simulink model "car_trailer_parking_model"  (R2024b)
settings: Solver=ode15s  StartTime=0.0  StopTime=5  FixedStep=1e-6  MaxStep=0.1  RelTol=1e-3  AbsTol=1e-6
undefined symbols (not defined in the file): Ion, Lithium, ref_traj_parking, ref_traj_reverse, ref_traj_straight
libraries: autolibshared x2, slpidlib x2, spsBatteryLib x1, spsDCMachineLib x1, spsGroundLib x1, spsFullBridgeMMCLib x1, spsPWMGenerator2LevelLib x1, vehdynlibeom x1, spsVariableCapacitorLib x1, spsVariableResistorLib x1, spspowerguiLib x1
(part 1 of 2)
settings Model: Creator=jesss  LastModifiedBy=jesss
settings SolverCC: MaxConsecutiveZCs=50  MaxConsecutiveMinStep=5  ZeroCrossControl=DisableAll
settings DataIOCC: SaveOutput=off  SignalLogging=off  SaveTime=off  ReturnWorkspaceOutputs=off
settings DebuggingCC: RTPrefix=none  StringTruncationChecking=none  AlgebraicLoopMsg=none  SignalResolutionControl=None  InheritedTsInSrcMsg=none  MultiTaskDSMMsg=none  MultiTaskCondExecSysMsg=none  MultiTaskRateTransMsg=warning  TasksWithSamePriorityMsg=none  SigSpecEnsureSampleTimeMsg=none  IntegerOverflowMsg=none  ParameterDowncastMsg=none  ParameterOverflowMsg=none  ParameterTunabilityLossMsg=none  FcnCallInpInsideContextMsg=warning  FrameProcessingCompatibilityMsg=none  UnknownTsInhSupMsg=none  NonCurrentReleaseOperatingPointMsg=warning  IntegerSaturationMsg=none
settings ModelReferenceCC: UpdateModelReferenceTargets=IfOutOfDate

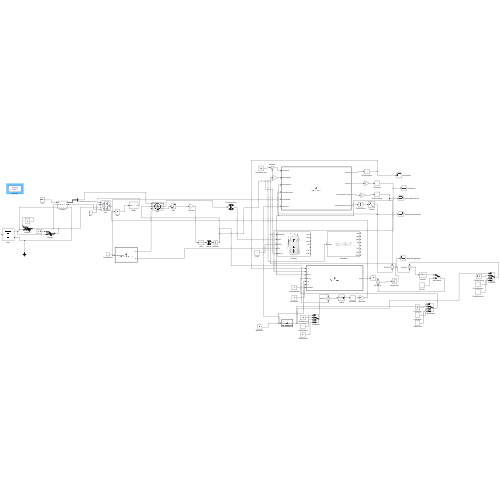
[thumbnail: Simulink's stored preview of the top-level diagram]
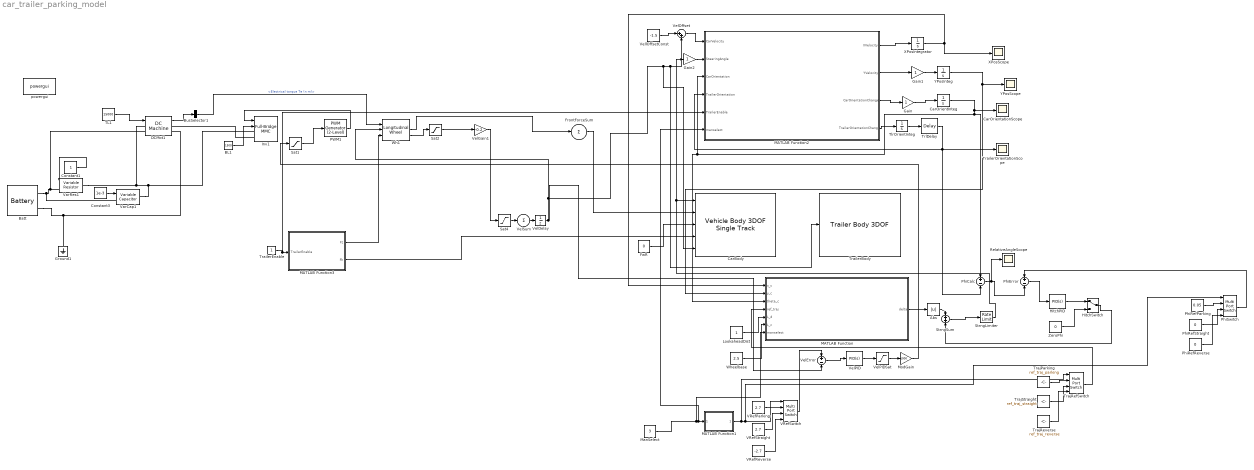
== system car_trailer_parking_model ==
  Abs : Abs  SaturateOnIntegerOverflow=off
  BL1 : Constant  Value=1500
  Batt : spsBatteryLib/Battery  BatType=Lithium-Ion  NomV=800  NomQ=100  SOC=100  Batt_Tr=0.01  PresetModel=on  MaxQ=100  MinV=600  FullV=931.1897  Dis_rate=43.4783  R=0.08  Normal_OP=90.4348  expZone="[864.3087      4.913043]"
  BusSelector1 : BusSelector  OutputSignals=Electrical torque Te (n m)
  CarBody : autolibshared/Vehicle Body 3DOF Single Track  trackMode=Single (bicycle)  inputMode=External longitudinal forces  frontSteerMode=on  rearSteerMode=off  windMode=off  muMode=off  extFMode=off  extMMode=off  htchFMode=on  htchMMode=off  extXo=off  extpsio=off  extxdoto=on  extro=off  extYo=off  extTamb=off  extydoto=off  aMode=2  NF=2  NR=2  m=3500  a=2  b=2  h=0.5  dh=1  hh=0.2  X_o=0  xdot_o=0  CalphaMode=off  sigmaMode=on  d=0  hl=0  w=[1.4,1.4]  Cy_f=100000  Cy_r=100000  sigma_f=0.3  sigma_r=0.3  alpha_f_brk=[-.1 .1]  Cy_f_data=[-9e3 9e3]  alpha_r_brk=[-.1 .1]  Cy_r_data=[-9e3 9e3]  Y_o=0  ydot_o=0  Izz=18667  psi_o=0  r_o=0  Af=2  Cd=0.3  Cl=0.1  Cpm=0  beta_w=[0 0.01:0.01:0.3]  Cs=[0 0.01:0.01:0.3]  Cym=[0 1e-6:0.01:0.3]  Pabs=101325  Tair=293  g=9.81  mu=0.8  xdot_tol=0.001  Fznom=8584  Fxtire_sat=7e4  Fytire_sat=7e4  longOff=0  latOff=0  vertOff=0  wrapAng=off
  CarOrientInteg : Integrator
  CarOrientationScope : Scope
  Constant1 : Constant
  Constant3 : Constant  Value=1e-3
  DCMot1 : spsDCMachineLib/DC Machine  PresetModel=No  MechanicalLoad=Torque TL  FieldType=Wound  ShowDetailedParameters=on  MeasurementBus=off  RLa="[0.8  0.01]"  RLf="[100  1]"  Laf=200  MachineConstant=Torque constant (N.m/A)  Ke=1.8  Kt=1.8  J=1000  Bm=0.01  Tf=0  w0=0  Ifinit=0  TsPowergui=0  TsBlock=-1
  FrontForceSum : Sum  Inputs=+
  FwR : Constant  Value=0
  Gain : Gain
  Gain1 : Gain
  Gain2 : Gain
  Ground1 : spsGroundLib/Ground  LConnTagsString=a
  HitchPID : slpidlib/PID Controller  Controller=PID  Form=Parallel  TimeDomain=Continuous-time  UseExternalTs=off  SampleTime=-1  IntegratorMethod=Forward Euler  FilterMethod=Forward Euler  ControllerParametersSource=internal  P=5  I=0.5  UseKiTs=off  D=0.05  UseExternalDerivativeSource=off  N=100  UseFilter=on  TunerSelectOption=Transfer Function Based (PID Tuner App)  InitialConditionSource=internal  InitialConditionForIntegrator=0  InitialConditionForFilter=0  DifferentiatorICPrevScaledInput=0  ExternalReset=none  TrackingMode=off  Kt=1  LimitOutput=off  SatLimitsSource=internal  UpperSaturationLimit=inf  LowerSaturationLimit=-inf  LinearizeAsGain=on  AntiWindupMode=none  Kb=1  LimitIntegrator=off  UpperIntegratorSaturationLimit=inf  LowerIntegratorSaturationLimit=-inf  POutMin=[]  POutMax=[]  IOutMin=[]  IOutMax=[]  DOutMin=[]  DOutMax=[]  NOutMin=[]  NOutMax=[]  SumOutMin=[]  SumOutMax=[]  SaturationOutMin=[]  SaturationOutMax=[]  PParamMin=[]  PParamMax=[]  IParamMin=[]  IParamMax=[]  DParamMin=[]  DParamMax=[]  NParamMin=[]  NParamMax=[]  KbParamMin=[]  KbParamMax=[]  KtParamMin=[]  KtParamMax=[]  KbOutMin=[]  KbOutMax=[]  KtOutMin=[]  KtOutMax=[]  IntegratorOutMin=[]  IntegratorOutMax=[]  FilterOutMin=[]  FilterOutMax=[]  SumI1OutMin=[]  SumI1OutMax=[]  SumI2OutMin=[]  SumI2OutMax=[]  SumI3OutMin=[]  SumI3OutMax=[]  SumI4OutMin=[]  SumI4OutMax=[]  SumDOutMin=[]  SumDOutMax=[]  DifferentiatorOutMin=[]  DifferentiatorOutMax=[]  FilterDiffOutCoefMin=[]  FilterDiffOutCoefMax=[]  ReciprocalOutMin=[]  ReciprocalOutMax=[]  SumDenOutMin=[]  SumDenOutMax=[]  SumNumOutMin=[]  SumNumOutMax=[]  DivideOutMin=[]  DivideOutMax=[]  UdiffTsProdOutMin=[]  UdiffTsProdOutMax=[]  NTsProdOutMin=[]  NTsProdOutMax=[]  UintegralTsProdOutMin=[]  UintegralTsProdOutMax=[]  UngainTsProdOutMin=[]  UngainTsProdOutMax=[]  ClampingZeroOutDataTypeStr=Inherit: Inherit via back propagation  ClampingZeroOutMin=[]  ClampingZeroOutMax=[]  FilterDenConstantOutDataTypeStr=Inherit: Inherit via back propagation  FilterDenConstantOutMin=[]  FilterDenConstantOutMax=[]  PCopyOutDataTypeStr=Inherit: Inherit via back propagation  PCopyOutMin=[]  PCopyOutMax=[]  NCopyOutDataTypeStr=Inherit: Inherit via back propagation  NCopyOutMin=[]  NCopyOutMax=[]  IntegratorContinuousStateAttributes=''  IntegratorStateMustResolveToSignalObject=off  IntegratorRTWStateStorageClass=Auto  FilterContinuousStateAttributes=''  FilterStateMustResolveToSignalObject=off  FilterRTWStateStorageClass=Auto  ParallelPVariant=InternalParameters  IdealPVariant=Disabled  IVariant=InternalParameters  DVariant=InternalParameters  IntegratorVariant=Continuous  SatVariant=Disabled  AWVariant=Passthrough  PCopyVariant=Disabled  TRVariant=Disabled  FdbkBlocksVariant=Forward  IdealPFdbkVariant=Disabled  SatFdbkVariant=Disabled  DerivativeFilterVariant=ContFilter  NVariant=InternalParameters  NCopyVariant=Disabled  FilterICVariant=InternalICsFilter  IntegratorICVariant=InternalICs  ExternalResetVariant=Disabled  TRSumVariant=Passthrough  SumFdbkVariant=Disabled  SumVariant=Sum_PID  TsampFilterVariant=InternalTs  TsampNgainVariant=Passthrough  TsampIntegralVariant=Disabled_SignalSpec  ExternalSaturationOutDataTypeStr=Inherit: Same as second input  DerivativeSourceVariant=ErrorSignal  PreIntVariant=InternalPreInt
  HitchSwitch : ManualSwitch
  Inv1 : spsFullBridgeMMCLib/Full-Bridge MMC  ModelType=Switching devices  n=1  C=1e-3  Vc_Initial=0  Ron=0.01  Rs=1e6  Cs=1e-9  Ron_Diode=1e-3  Rs_Diode=1e6  Cs_Diode=inf  Vf_Diode=1e-3  Rs_CurrentSource=inf  Ts=10e-6
      settings: LibrarySourceBlock=sps_lib/Power Electronics/Full-Bridge MMC
  LookaheadDist : Constant
  MATLAB Function : MATLAB Function  TreatAsAtomicUnit=on
  MATLAB Function1 : MATLAB Function  TreatAsAtomicUnit=on
  MATLAB Function2 : MATLAB Function  TreatAsAtomicUnit=on
  MATLAB Function3 : MATLAB Function  TreatAsAtomicUnit=on
  ManSelect : Constant  Value=3
  ModGain : Gain  Gain=1000
  PWM1 : spsPWMGenerator2LevelLib/PWM Generator (2-Level)  ModulatorType=Single-phase full-bridge (4 pulses)  ModulatorMode=Unsynchronized  Fc=10000  Pc=0  nF=27  MinMax=[-1, 1]  SamplingTechnique=Symmetrical regular (single edge)  ModulatingSignals=off  m=0.8  Freq=60  Phase=0  Ts=1e-5  ShowCarrierOutport=off
  PhiCalc : Sum  Inputs=+-
  PhiError : Sum  Inputs=+-
  PhiRefParking : Constant  Value=0.05
  PhiRefReverse : Constant  Value=0
  PhiRefStraight : Constant  Value=0
  PhiSwitch : MultiPortSwitch  SaturateOnIntegerOverflow=off  InputSameDT=off
  RelativeAngleScope : Scope
  Sat1 : Saturate  UpperLimit=50000  LowerLimit=-50000
  Sat2 : Saturate  UpperLimit=6  LowerLimit=-6
  Sat4 : Saturate  UpperLimit=2.5  LowerLimit=-2.5
  StrngLimiter : RateLimiter  RisingSlewLimit=0.5  FallingSlewLimit=-0.5  SampleTimeMode=inherited
  StrngSum : Sum
  TL1 : Constant  Value=15000
  TlrOrientInteg : Integrator
  TrailerBody : vehdynlibeom/Trailer Body 3DOF  trackMode=Dual 2-axle  inputMode=External longitudinal velocity  frontSteerMode=off  middleSteerMode=off  rearSteerMode=off  windMode=off  muMode=off  extFMode=off  extMMode=off  FhtchFMode=off  FhtchMMode=off  RhtchFMode=off  RhtchMMode=off  extXo=off  extpsio=off  extxdoto=off  extro=off  extYo=off  extTamb=off  extydoto=off  aMode=2  NF=1  NM=2  NR=2  m=10000  a=3  b=4.5  c=3  h=0.5  dh_f=7.5  hh_f=0.6  dh_r=7.5  hh_r=0.6  X_o=0  xdot_o=0  Lcpm=0  CalphaMode=off  sigmaMode=on  d=0  hl_f=0  hl_r=0  w_f=0.1  w_m=1.82  w_r=2  w=[0.1 2]  Cy_f=1000  Cy_m=11e3  Cy_r=150000  sigma_f=0.1  sigma_m=.1  sigma_r=0.3  alpha_f_brk=[-.1 .1]  Cy_f_data=[-9e3 9e3]  alpha_m_brk=[-.1 .1]  Cy_m_data=[-9e3 9e3]  alpha_r_brk=[-.1 .1]  Cy_r_data=[-9e3 9e3]  Y_o=0  ydot_o=0  Izz=30000  psi_o=0  r_o=0  Af=3  Cd=0.4  Cl=0.1  Cpm=0  beta_w=[0:0.01:0.3]  Cs=[0:0.03:0.9]  Cym=[0:0.01:0.3]  Pabs=101325  Tair=293  g=9.81  mu=0.8  xdot_tol=0.001  Fznom=32700  Fxtire_sat=7e4  Fytire_sat=7e4  longOff=0  latOff=0  vertOff=0  wrapAng=off
  TrailerEnable : Constant
  TrailerOrientationScope : Scope
  TrajParking : Constant  Value=ref_traj_parking
  TrajRefSwitch : MultiPortSwitch  SaturateOnIntegerOverflow=off  InputSameDT=off
  TrajReverse : Constant  Value=ref_traj_reverse
  TrajStraight : Constant  Value=ref_traj_straight
  TrlDelay : TransportDelay  DelayTime=0.01  BufferSize=10240
  VRefParking : Constant  Value=2.7
  VRefReverse : Constant  Value=-2.7
  VRefStraight : Constant  Value=2.7
  VRefSwitch : MultiPortSwitch  SaturateOnIntegerOverflow=off  InputSameDT=off
  VarCap1 : spsVariableCapacitorLib/Variable Capacitor  methode=Backward Euler  Cabsmin=1e-9  Initialize=off  vC0=0  C0=1e-6  iC0=0
      settings: LibrarySourceBlock=sps_lib/Passives/Variable Capacitor
  VarRes1 : spsVariableResistorLib/Variable Resistor  Rabsmin=1e-6
      settings: LibrarySourceBlock=sps_lib/Passives/Variable Resistor
  VelDelay : UnitDelay  SampleTime=1e-3  HasFrameUpgradeWarning=on
  VelError : Sum  Inputs=+-
  VelGain1 : Gain  Gain=-0.2
  VelOffset : Sum  Inputs=|++
  VelPID : slpidlib/PID Controller  Controller=PID  Form=Parallel  TimeDomain=Continuous-time  UseExternalTs=off  SampleTime=-1  IntegratorMethod=Forward Euler  FilterMethod=Forward Euler  ControllerParametersSource=internal  P=500  I=0.1  UseKiTs=off  D=0.2  UseExternalDerivativeSource=off  N=100  UseFilter=on  TunerSelectOption=Transfer Function Based (PID Tuner App)  InitialConditionSource=internal  InitialConditionForIntegrator=0  InitialConditionForFilter=0  DifferentiatorICPrevScaledInput=0  ExternalReset=none  TrackingMode=off  Kt=1  LimitOutput=on  SatLimitsSource=internal  UpperSaturationLimit=inf  LowerSaturationLimit=-inf  LinearizeAsGain=on  AntiWindupMode=back-calculation  Kb=1  LimitIntegrator=off  UpperIntegratorSaturationLimit=inf  LowerIntegratorSaturationLimit=-inf  POutMin=[]  POutMax=[]  IOutMin=[]  IOutMax=[]  DOutMin=[]  DOutMax=[]  NOutMin=[]  NOutMax=[]  SumOutMin=[]  SumOutMax=[]  SaturationOutMin=[]  SaturationOutMax=[]  PParamMin=[]  PParamMax=[]  IParamMin=[]  IParamMax=[]  DParamMin=[]  DParamMax=[]  NParamMin=[]  NParamMax=[]  KbParamMin=[]  KbParamMax=[]  KtParamMin=[]  KtParamMax=[]  KbOutMin=[]  KbOutMax=[]  KtOutMin=[]  KtOutMax=[]  IntegratorOutMin=[]  IntegratorOutMax=[]  FilterOutMin=[]  FilterOutMax=[]  SumI1OutMin=[]  SumI1OutMax=[]  SumI2OutMin=[]  SumI2OutMax=[]  SumI3OutMin=[]  SumI3OutMax=[]  SumI4OutMin=[]  SumI4OutMax=[]  SumDOutMin=[]  SumDOutMax=[]  DifferentiatorOutMin=[]  DifferentiatorOutMax=[]  FilterDiffOutCoefMin=[]  FilterDiffOutCoefMax=[]  ReciprocalOutMin=[]  ReciprocalOutMax=[]  SumDenOutMin=[]  SumDenOutMax=[]  SumNumOutMin=[]  SumNumOutMax=[]  DivideOutMin=[]  DivideOutMax=[]  UdiffTsProdOutMin=[]  UdiffTsProdOutMax=[]  NTsProdOutMin=[]  NTsProdOutMax=[]  UintegralTsProdOutMin=[]  UintegralTsProdOutMax=[]  UngainTsProdOutMin=[]  UngainTsProdOutMax=[]  ClampingZeroOutDataTypeStr=Inherit: Inherit via back propagation  ClampingZeroOutMin=[]  ClampingZeroOutMax=[]  FilterDenConstantOutDataTypeStr=Inherit: Inherit via back propagation  FilterDenConstantOutMin=[]  FilterDenConstantOutMax=[]  PCopyOutDataTypeStr=Inherit: Inherit via back propagation  PCopyOutMin=[]  PCopyOutMax=[]  NCopyOutDataTypeStr=Inherit: Inherit via back propagation  NCopyOutMin=[]  NCopyOutMax=[]  IntegratorContinuousStateAttributes=''  IntegratorStateMustResolveToSignalObject=off  IntegratorRTWStateStorageClass=Auto  FilterContinuousStateAttributes=''  FilterStateMustResolveToSignalObject=off  FilterRTWStateStorageClass=Auto  ParallelPVariant=InternalParameters  IdealPVariant=Disabled  IVariant=InternalParameters  DVariant=InternalParameters  IntegratorVariant=Continuous  SatVariant=Enabled  AWVariant=BackCalculation  PCopyVariant=Disabled  TRVariant=Disabled  FdbkBlocksVariant=Forward  IdealPFdbkVariant=Disabled  SatFdbkVariant=Disabled  DerivativeFilterVariant=ContFilter  NVariant=InternalParameters  NCopyVariant=Disabled  FilterICVariant=InternalICsFilter  IntegratorICVariant=InternalICs  ExternalResetVariant=Disabled  TRSumVariant=Passthrough  SumFdbkVariant=Disabled  SumVariant=Sum_PID  TsampFilterVariant=InternalTs  TsampNgainVariant=Passthrough  TsampIntegralVariant=Disabled_SignalSpec  ExternalSaturationOutDataTypeStr=Inherit: Same as second input  DerivativeSourceVariant=ErrorSignal  PreIntVariant=InternalPreInt
  VelPIDSat : Saturate  UpperLimit=50  LowerLimit=-50
  VelSum : Sum  Inputs=+
  VellOffsetConst : Constant  Value=-1.5
  Wh1 : autolibshared/Longitudinal Wheel  FxType=Magic Formula constant value  rollingType=None  BrakeType=None  vertType=None  lam_x=1  extMu=off  aMode=2  br=0  Iyy=5000  omegao=0  Lrel=0.3  Re=0.3  UNLOADED_RADIUS=0.4  LONGVL=16  gamma=0  NOMPRES=220000  press=220000  extPress=off  Dx=1  Cx=1.5  Bx=15  Ex=2  PCX1=1.6  PDX1=1  PDX2=-0.08  PDX3=0  PEX1=0.112  PEX2=0.313  PEX3=0  PEX4=0.0016  PKX1=21.7  PKX2=13.77  PKX3=-0.412  PHX1=2.1585E-4  PHX2=0.00115  PVX1=1.5973E-5  PVX2=1.043E-4  PPX1=-0.3489  PPX2=0.382  PPX3=-0.09634  PPX4=0.06447  lam_muV=1  lam_Kxkappa=1  lam_Cx=1  lam_Ex=0  lam_Hx=1  lam_Vx=1  kappaFx=[-1,-0.78476,-0.61585,-0.48329,-0.37927,-0.29764,-0.23357,-0.1833,-0.14384,-0.11288,-0.088587,-0.069519,-0.054556,-0.042813,-0.033598,-0.026367,-0.020691,-0.016238,-0.012743,-0.01,0.01,0.012743,0.016238,0.020691,0.026367,0.033598,0.042813,0.054556,0.069519,0.088587,0.11288,0.14384,0.1833,0.23357,0.29764,0.37927,0.48329,0.61585,0.78476,1]  FzFx=[0,200,400,600,800,1000,1200,1400,1600,1800,2000,2200,2400,2600,2800,3000,3200,3400,3600,3800,4000,4200,4400,4600,4800,5000,5200,5400,5600,5800,6000,6200,6400,6600,6800,7000,7200,7400,7600,7800,8000,8200,8400,8600,8800,9000,9200,9400,9600,9800,10000]  FxMap=|  aMy=84e-4  bMy=6.2e-4  cMy=1.6e-4  alphaMy=-0.003  betaMy=0.97  QSY1=0.007  QSY2=0  QSY3=0.0015  QSY4=8.5e-05  QSY5=0  QSY6=0  QSY7=0.9  QSY8=-0.4  lam_My=1  VxMy=-20:1:20  FzMy=0:200:1e4  MyMap=|  Fpl=10  Cr=1e-3  Kt=.008  Tmeas=25  Tamb=298.15  extTamb=off  mu_static=0.3  mu_kinetic=0.2  disk_abore=0.05  Rm=0.1778  num_pads=2  drum_abore=0.0508  drum_a=0.123  drum_c=0.212  drum_r=0.15  drum_theta1=0  drum_theta2=126  brake_p_bpt=[1 11.4736842105263 21.9473684210526 32.4210526315789 42.8947368421053 53.3684210526316 63.8421052631579 74.3157894736842 84.7894736842105 95.2631578947368 105.736842105263 116.210526315789 126.684210526316 137.157894736842 147.631578947368 158.105263157895 168.578947368421 179.052631578947 189.526315789474 200]  brake_n_bpt=[0 52.6315789473684 105.263157894737 157.894736842105 210.526315789474 263.157894736842 315.789473684211 368.421052631579 421.052631578947 473.684210526316 526.315789473684 578.947368421053 631.578947368421 684.210526315789 736.842105263158 789.473684210526 842.105263157895 894.736842105263 947.368421052632 1000]  f_brake_t=[43.4900602404453 42.5056030554862 41.5350898940194 40.5780454442085 39.6340111501808 38.7025443887544 37.7832176914519 36.8756180088306 35.9793460143796 35.0940154454303 34.2192524787115 33.3546951383474 32.4999927342521 31.6548053290159 30.8188032315107 29.991666515561 29.1730845621415 28.362755623661 27.5603864089927 26.765691687993;498.991217495636 487.695866636631 476.560505099801 465.579679307235 454.748127933653 444.060772460445 433.51270824929 423.099196101319 412.81565427025 402.657650900201 392.620896861006 382.701238955775 372.894653477208 363.197240090814 353.605216024701 344.114910546964 334.722759712992 325.425301366216 316.219170376863 307.10109410434;954.492374750826 932.886130217776 911.585920305583 890.581313170261 869.862244717126 849.419000532136 829.242198807128 809.322774193808 789.651962526121 770.221286354971 751.0225412433 732.047782773203 713.289314220164 694.739674852612 676.391628817892 658.238154578366 640.272434863842 622.48784710877 604.877954344734 587.436496520688;1409.99353200602 1378.07639379892 1346.61133551136 1315.58294703329 1284.9763615006 1254.77722860383 1224.97168936497 1195.5463522863 1166.48827078199 1137.78492180974 1109.42418562559 1081.39432659063 1053.68397496312 1026.28210961441 999.178041611083 972.361398609768 945.822110014692 919.550392851325 893.536738312604 867.771898937035;1865.49468926121 1823.26665738007 1781.63675071715 1740.58458089631 1700.09047828407 1660.13545667552 1620.7011799228 1581.76993037878 1543.32457903786 1505.34855726451 1467.82583000789 1430.74087040806 1394.07863570608 1357.82454437621 1321.96445440427 1286.48464264117 1251.37178516554 1216.61293859388 1182.19552228048 1148.10730135338;2320.9958465164 2268.45692096121 2216.66216592293 2165.58621475934 2115.20459506754 2065.49368474721 2016.43067048064 1967.99350847127 1920.16088729373 1872.91219271928 1826.22747439018 1780.08741422549 1734.47329644903 1689.36697913801 1644.75086719747 1600.60788667257 1556.92146031639 1513.67548433643 1470.85430624835 1428.44270376973;2776.49700377159 2713.64718454235 2651.68758112871 2590.58784862237 2530.31871185102 2470.8519128189 2412.16016103848 2354.21708656376 2296.9971955496 2240.47582817405 2184.62911877248 2129.43395804292 2074.86795719199 2020.9094138998 1967.53727999066 1914.73113070398 1862.47113546724 1810.73803007899 1759.51309021622 1708.77810618608;3231.99816102678 3158.8374481235 3086.71299633449 3015.58948248539 2945.43282863449 2876.21014089059 2807.88965159632 2740.44066465625 2673.83350380547 2608.03946362882 2543.03076315477 2478.78050186034 2415.26261793494 2352.4518486616 2290.32369278385 2228.85437473538 2168.02081061809 2107.80057582154 2048.17187418409 1989.11350860242;3687.49931828197 3604.02771170464 3521.73841154027 3440.59111634842 3360.54694541796 3281.56836896228 3203.61914215416 3126.66424274874 3050.66981206134 2975.60309908359 2901.43240753707 2828.12704567777 2755.6572786779 2683.9942834234 2613.11010557704 2542.97761876678 2473.57048576894 2404.8631215641 2336.83065815196 2269.44891101877;4143.00047553716 4049.21797528579 3956.76382674606 3865.59275021144 3775.66106220143 3686.92659703397 3599.34863271199 3512.88782084123 3427.50612031721 3343.16673453836 3259.83405191936 3177.4735894952 3096.05193942085 3015.5367181852 2935.89651837023 2857.10086279818 2779.12016091979 2701.92566730665 2625.48944211983 2549.78431343512;4598.50163279235 4494.40823886693 4391.78924195184 4290.59438407447 4190.77517898491 4092.28482510566 3995.07812326983 3899.11139893372 3804.34242857308 3710.73036999313 3618.23569630166 3526.82013331263 3436.44660016381 3347.079152947 3258.68293116342 3171.22410682959 3084.66983607064 2998.98821304921 2914.1482260877 2830.11971585147;5054.00279004754 4939.59850244808 4826.81465715762 4715.59601793749 4605.88929576838 4497.64305317735 4390.80761382767 4285.3349770262 4181.17873682896 4078.2940054479 3976.63734068395 3876.16667713006 3776.84126090677 3678.62158770879 3581.46934395661 3485.34735086099 ...(+2764 chars)]  FNOMIN=2000  lam_Fzo=1  m=10  zo=0  zdoto=0  g=9.81  VERTICAL_STIFFNESS=209000.0  VERTICAL_DAMPING=50  Q_RE0=.99  Q_V1=0  Q_V2=0.047  Q_FZ1=0  Q_FZ2=15.4  Q_FCX=0.134  Q_FCY=.11  Q_CAM=0  PFZ1=0.71  Q_FCY2=-0.48  Q_CAM1=85.2  Q_CAM2=257.0  Q_CAM3=0.512  Q_FYS1=-204500.0  Q_FYS2=-60000  Q_FYS3=88211.7  BOTTOM_OFFST=.01  BOTTOM_STIFF=2000000  zFz=[0 .01 .1]  pFz=[10000 1000000]  Fzz=[0 1e3 1e4; 0 1e4 1e5]  zdotFz=[-20 0 20]  Fzzdot=[500 0 -500;250 0 -250]  Gndz=0  extGnd=off  FZMIN=1000  FZMAX=50000  PRESMIN=10000  PRESMAX=1000000  kappamax=0.005  VXLOW=0.01  TMIN=0  TMAX=400  blkID=0
      FxMap=|
      | [-0,-131.22,-262.44,-393.66,-524.88,-656.1,-787.32,-918.54,-1049.8,-1181,-1312.2,-1443.4,-1574.6,-1705.9,-1837.1,-1968.3,-2099.5,-2230.7,-2362,-2493.2,-2624.4,-2755.6,-2886.8,-3018.1,-3149.3,-3280.5,-3411.7,-3542.9,-3674.2,-3805.4,-3936.6,-4067.8,-4199,-4330.2,-4461.5,-4592.7,-4723.9,-4855.1,-4986.3,-5117.6,-5248.8,-5380,-5511.2,-5642.4,-5773.7,-5904.9,-6036.1,-6167.3,-6298.5,-6429.8,-6561
      | -0,-137.87,-275.75,-413.62,-551.49,-689.36,-827.24,-965.11,-1103,-1240.9,-1378.7,-1516.6,-1654.5,-1792.3,-1930.2,-2068.1,-2206,-2343.8,-2481.7,-2619.6,-2757.5,-2895.3,-3033.2,-3171.1,-3308.9,-3446.8,-3584.7,-3722.6,-3860.4,-3998.3,-4136.2,-4274,-4411.9,-4549.8,-4687.7,-4825.5,-4963.4,-5101.3,-5239.2,-5377,-5514.9,-5652.8,-5790.6,-5928.5,-6066.4,-6204.3,-6342.1,-6480,-6617.9,-6755.8,-6893.6
      | -0,-145.88,-291.75,-437.63,-583.5,-729.38,-875.25,-1021.1,-1167,-1312.9,-1458.8,-1604.6,-1750.5,-1896.4,-2042.3,-2188.1,-2334,-2479.9,-2625.8,-2771.6,-2917.5,-3063.4,-3209.3,-3355.1,-3501,-3646.9,-3792.8,-3938.6,-4084.5,-4230.4,-4376.3,-4522.1,-4668,-4813.9,-4959.8,-5105.6,-5251.5,-5397.4,-5543.3,-5689.1,-5835,-5980.9,-6126.8,-6272.6,-6418.5,-6564.4,-6710.3,-6856.1,-7002,-7147.9,-7293.8
      | -0,-155.26,-310.53,-465.79,-621.05,-776.32,-931.58,-1086.8,-1242.1,-1397.4,-1552.6,-1707.9,-1863.2,-2018.4,-2173.7,-2328.9,-2484.2,-2639.5,-2794.7,-2950,-3105.3,-3260.5,-3415.8,-3571.1,-3726.3,-3881.6,-4036.8,-4192.1,-4347.4,-4502.6,-4657.9,-4813.2,-4968.4,-5123.7,-5278.9,-5434.2,-5589.5,-5744.7,-5900,-6055.3,-6210.5,-6365.8,-6521.1,-6676.3,-6831.6,-6986.8,-7142.1,-7297.4,-7452.6,-7607.9,-7763.2
      | -0,-165.86,-331.71,-497.57,-663.43,-829.28,-995.14,-1161,-1326.9,-1492.7,-1658.6,-1824.4,-1990.3,-2156.1,-2322,-2487.8,-2653.7,-2819.6,-2985.4,-3151.3,-3317.1,-3483,-3648.8,-3814.7,-3980.6,-4146.4,-4312.3,-4478.1,-4644,-4809.8,-4975.7,-5141.5,-5307.4,-5473.3,-5639.1,-5805,-5970.8,-6136.7,-6302.5,-6468.4,-6634.3,-6800.1,-6966,-7131.8,-7297.7,-7463.5,-7629.4,-7795.2,-7961.1,-8127,-8292.8
      | -0,-177.09,-354.19,-531.28,-708.38,-885.47,-1062.6,-1239.7,-1416.8,-1593.8,-1770.9,-1948,-2125.1,-2302.2,-2479.3,-2656.4,-2833.5,-3010.6,-3187.7,-3364.8,-3541.9,-3719,-3896.1,-4073.2,-4250.3,-4427.4,-4604.5,-4781.5,-4958.6,-5135.7,-5312.8,-5489.9,-5667,-5844.1,-6021.2,-6198.3,-6375.4,-6552.5,-6729.6,-6906.7,-7083.8,-7260.9,-7438,-7615.1,-7792.1,-7969.2,-8146.3,-8323.4,-8500.5,-8677.6,-8854.7
      | -0,-187.84,-375.67,-563.51,-751.35,-939.18,-1127,-1314.9,-1502.7,-1690.5,-1878.4,-2066.2,-2254,-2441.9,-2629.7,-2817.5,-3005.4,-3193.2,-3381.1,-3568.9,-3756.7,-3944.6,-4132.4,-4320.2,-4508.1,-4695.9,-4883.7,-5071.6,-5259.4,-5447.3,-5635.1,-5822.9,-6010.8,-6198.6,-6386.4,-6574.3,-6762.1,-6949.9,-7137.8,-7325.6,-7513.5,-7701.3,-7889.1,-8077,-8264.8,-8452.6,-8640.5,-8828.3,-9016.1,-9204,-9391.8
      | -0,-196.25,-392.49,-588.74,-784.98,-981.23,-1177.5,-1373.7,-1570,-1766.2,-1962.5,-2158.7,-2354.9,-2551.2,-2747.4,-2943.7,-3139.9,-3336.2,-3532.4,-3728.7,-3924.9,-4121.2,-4317.4,-4513.6,-4709.9,-4906.1,-5102.4,-5298.6,-5494.9,-5691.1,-5887.4,-6083.6,-6279.9,-6476.1,-6672.3,-6868.6,-7064.8,-7261.1,-7457.3,-7653.6,-7849.8,-8046.1,-8242.3,-8438.6,-8634.8,-8831,-9027.3,-9223.5,-9419.8,-9616,-9812.3
      | -0,-199.97,-399.95,-599.92,-799.9,-999.87,-1199.8,-1399.8,-1599.8,-1799.8,-1999.7,-2199.7,-2399.7,-2599.7,-2799.6,-2999.6,-3199.6,-3399.6,-3599.5,-3799.5,-3999.5,-4199.5,-4399.4,-4599.4,-4799.4,-4999.4,-5199.3,-5399.3,-5599.3,-5799.2,-5999.2,-6199.2,-6399.2,-6599.1,-6799.1,-6999.1,-7199.1,-7399,-7599,-7799,-7999,-8198.9,-8398.9,-8598.9,-8798.9,-8998.8,-9198.8,-9398.8,-9598.8,-9798.7,-9998.7
      | -0,-196.87,-393.74,-590.6,-787.47,-984.34,-1181.2,-1378.1,-1574.9,-1771.8,-1968.7,-2165.5,-2362.4,-2559.3,-2756.2,-2953,-3149.9,-3346.8,-3543.6,-3740.5,-3937.4,-4134.2,-4331.1,-4528,-4724.8,-4921.7,-5118.6,-5315.4,-5512.3,-5709.2,-5906,-6102.9,-6299.8,-6496.6,-6693.5,-6890.4,-7087.2,-7284.1,-7481,-7677.8,-7874.7,-8071.6,-8268.5,-8465.3,-8662.2,-8859.1,-9055.9,-9252.8,-9449.7,-9646.5,-9843.4
      | -0,-186.02,-372.04,-558.06,-744.08,-930.1,-1116.1,-1302.1,-1488.2,-1674.2,-1860.2,-2046.2,-2232.2,-2418.3,-2604.3,-2790.3,-2976.3,-3162.3,-3348.4,-3534.4,-3720.4,-3906.4,-4092.4,-4278.5,-4464.5,-4650.5,-4836.5,-5022.5,-5208.6,-5394.6,-5580.6,-5766.6,-5952.6,-6138.7,-6324.7,-6510.7,-6696.7,-6882.7,-7068.7,-7254.8,-7440.8,-7626.8,-7812.8,-7998.8,-8184.9,-8370.9,-8556.9,-8742.9,-8928.9,-9115,-9301
      | -0,-168.44,-336.89,-505.33,-673.78,-842.22,-1010.7,-1179.1,-1347.6,-1516,-1684.4,-1852.9,-2021.3,-2189.8,-2358.2,-2526.7,-2695.1,-2863.5,-3032,-3200.4,-3368.9,-3537.3,-3705.8,-3874.2,-4042.7,-4211.1,-4379.5,-4548,-4716.4,-4884.9,-5053.3,-5221.8,-5390.2,-5558.6,-5727.1,-5895.5,-6064,-6232.4,-6400.9,-6569.3,-6737.8,-6906.2,-7074.6,-7243.1,-7411.5,-7580,-7748.4,-7916.9,-8085.3,-8253.7,-8422.2
      | -0,-146.7,-293.4,-440.1,-586.81,-733.51,-880.21,-1026.9,-1173.6,-1320.3,-1467,-1613.7,-1760.4,-1907.1,-2053.8,-2200.5,-2347.2,-2493.9,-2640.6,-2787.3,-2934,-3080.7,-3227.4,-3374.1,-3520.8,-3667.5,-3814.2,-3960.9,-4107.6,-4254.3,-4401,-4547.7,-4694.5,-4841.2,-4987.9,-5134.6,-5281.3,-5428,-5574.7,-5721.4,-5868.1,-6014.8,-6161.5,-6308.2,-6454.9,-6601.6,-6748.3,-6895,-7041.7,-7188.4,-7335.1
      | -0,-123.75,-247.49,-371.24,-494.99,-618.73,-742.48,-866.23,-989.98,-1113.7,-1237.5,-1361.2,-1485,-1608.7,-1732.5,-1856.2,-1980,-2103.7,-2227.4,-2351.2,-2474.9,-2598.7,-2722.4,-2846.2,-2969.9,-3093.7,-3217.4,-3341.2,-3464.9,-3588.7,-3712.4,-3836.2,-3959.9,-4083.7,-4207.4,-4331.1,-4454.9,-4578.6,-4702.4,-4826.1,-4949.9,-5073.6,-5197.4,-5321.1,-5444.9,-5568.6,-5692.4,-5816.1,-5939.9,-6063.6,-6187.3
      | -0,-101.91,-203.81,-305.72,-407.63,-509.53,-611.44,-713.35,-815.25,-917.16,-1019.1,-1121,-1222.9,-1324.8,-1426.7,-1528.6,-1630.5,-1732.4,-1834.3,-1936.2,-2038.1,-2140,-2241.9,-2343.9,-2445.8,-2547.7,-2649.6,-2751.5,-2853.4,-2955.3,-3057.2,-3159.1,-3261,-3362.9,-3464.8,-3566.7,-3668.6,-3770.5,-3872.5,-3974.4,-4076.3,-4178.2,-4280.1,-4382,-4483.9,-4585.8,-4687.7,-4789.6,-4891.5,-4993.4,-5095.3
      | -0,-82.514,-165.03,-247.54,-330.06,-412.57,-495.09,-577.6,-660.12,-742.63,-825.14,-907.66,-990.17,-1072.7,-1155.2,-1237.7,-1320.2,-1402.7,-1485.3,-1567.8,-1650.3,-1732.8,-1815.3,-1897.8,-1980.3,-2062.9,-2145.4,-2227.9,-2310.4,-2392.9,-2475.4,-2557.9,-2640.5,-2723,-2805.5,-2888,-2970.5,-3053,-3135.6,-3218.1,-3300.6,-3383.1,-3465.6,-3548.1,-3630.6,-3713.2,-3795.7,-3878.2,-3960.7,-4043.2,-4125.7
      | -0,-66.058,-132.12,-198.17,-264.23,-330.29,-396.35,-462.41,-528.46,-594.52,-660.58,-726.64,-792.7,-858.76,-924.81,-990.87,-1056.9,-1123,-1189,-1255.1,-1321.2,-1387.2,-1453.3,-1519.3,-1585.4,-1651.5,-1717.5,-1783.6,-1849.6,-1915.7,-1981.7,-2047.8,-2113.9,-2179.9,-2246,-2312,-2378.1,-2444.2,-2510.2,-2576.3,-2642.3,-2708.4,-2774.4,-2840.5,-2906.6,-2972.6,-3038.7,-3104.7,-3170.8,-3236.8,-3302.9
      | -0,-52.494,-104.99,-157.48,-209.98,-262.47,-314.97,-367.46,-419.95,-472.45,-524.94,-577.44,-629.93,-682.43,-734.92,-787.41,-839.91,-892.4,-944.9,-997.39,-1049.9,-1102.4,-1154.9,-1207.4,-1259.9,-1312.4,-1364.9,-1417.3,-1469.8,-1522.3,-1574.8,-1627.3,-1679.8,-1732.3,-1784.8,-1837.3,-1889.8,-1942.3,-1994.8,-2047.3,-2099.8,-2152.3,-2204.8,-2257.3,-2309.7,-2362.2,-2414.7,-2467.2,-2519.7,-2572.2,-2624.7
      | -0,-41.519,-83.039,-124.56,-166.08,-207.6,-249.12,-290.64,-332.15,-373.67,-415.19,-456.71,-498.23,-539.75,-581.27,-622.79,-664.31,-705.83,-747.35,-788.87,-830.39,-871.91,-913.42,-954.94,-996.46,-1038,-1079.5,-1121,-1162.5,-1204.1,-1245.6,-1287.1,-1328.6,-1370.1,-1411.7,-1453.2,-1494.7,-1536.2,-1577.7,-1619.3,-1660.8,-1702.3,-1743.8,-1785.3,-1826.8,-1868.4,-1909.9,-1951.4,-1992.9,-2034.4,-2076
      | -0,-32.742,-65.483,-98.225,-130.97,-163.71,-196.45,-229.19,-261.93,-294.67,-327.42,-360.16,-392.9,-425.64,-458.38,-491.12,-523.86,-556.61,-589.35,-622.09,-654.83,-687.57,-720.31,-753.06,-785.8,-818.54,-851.28,-884.02,-916.76,-949.5,-982.25,-1015,-1047.7,-1080.5,-1113.2,-1146,-1178.7,-1211.4,-1244.2,-1276.9,-1309.7,-1342.4,-1375.1,-1407.9,-1440.6,-1473.4,-1506.1,-1538.9,-1571.6,-1604.3,-1637.1
      | 0,32.742,65.483,98.225,130.97,163.71,196.45,229.19,261.93,294.67,327.42,360.16,392.9,425.64,458.38,491.12,523.86,556.61,589.35,622.09,654.83,687.57,720.31,753.06,785.8,818.54,851.28,884.02,916.76,949.5,982.25,1015,1047.7,1080.5,1113.2,1146,1178.7,1211.4,1244.2,1276.9,1309.7,1342.4,1375.1,1407.9,1440.6,1473.4,1506.1,1538.9,1571.6,1604.3,1637.1
      | 0,41.519,83.039,124.56,166.08,207.6,249.12,290.64,332.15,373.67,415.19,456.71,498.23,539.75,581.27,622.79,664.31,705.83,747.35,788.87,830.39,871.91,913.42,954.94,996.46,1038,1079.5,1121,1162.5,1204.1,1245.6,1287.1,1328.6,1370.1,1411.7,1453.2,1494.7,1536.2,1577.7,1619.3,1660.8,1702.3,1743.8,1785.3,1826.8,1868.4,1909.9,1951.4,1992.9,2034.4,2076
      | 0,52.494,104.99,157.48,209.98,262.47,314.97,367.46,419.95,472.45,524.94,577.44,629.93,682.43,734.92,787.41,839.91,892.4,944.9,997.39,1049.9,1102.4,1154.9,1207.4,1259.9,1312.4,1364.9,1417.3,1469.8,1522.3,1574.8,1627.3,1679.8,1732.3,1784.8,1837.3,1889.8,1942.3,1994.8,2047.3,2099.8,2152.3,2204.8,2257.3,2309.7,2362.2,2414.7,2467.2,2519.7,2572.2,2624.7
      | 0,66.058,132.12,198.17,264.23,330.29,396.35,462.41,528.46,594.52,660.58,726.64,792.7,858.76,924.81,990.87,1056.9,1123,1189,1255.1,1321.2,1387.2,1453.3,1519.3,1585.4,1651.5,1717.5,1783.6,1849.6,1915.7,1981.7,2047.8,2113.9,2179.9,2246,2312,2378.1,2444.2,2510.2,2576.3,2642.3,2708.4,2774.4,2840.5,2906.6,2972.6,3038.7,3104.7,3170.8,3236.8,3302.9
      | 0,82.514,165.03,247.54,330.06,412.57,495.09,577.6,660.12,742.63,825.14,907.66,990.17,1072.7,1155.2,1237.7,1320.2,1402.7,1485.3,1567.8,1650.3,1732.8,1815.3,1897.8,1980.3,2062.9,2145.4,2227.9,2310.4,2392.9,2475.4,2557.9,2640.5,2723,2805.5,2888,2970.5,3053,3135.6,3218.1,3300.6,3383.1,3465.6,3548.1,3630.6,3713.2,3795.7,3878.2,3960.7,4043.2,4125.7
      | 0,101.91,203.81,305.72,407.63,509.53,611.44,713.35,815.25,917.16,1019.1,1121,1222.9,1324.8,1426.7,1528.6,1630.5,1732.4,1834.3,1936.2,2038.1,2140,2241.9,2343.9,2445.8,2547.7,2649.6,2751.5,2853.4,2955.3,3057.2,3159.1,3261,3362.9,3464.8,3566.7,3668.6,3770.5,3872.5,3974.4,4076.3,4178.2,4280.1,4382,4483.9,4585.8,4687.7,4789.6,4891.5,4993.4,5095.3
      | 0,123.75,247.49,371.24,494.99,618.73,742.48,866.23,989.98,1113.7,1237.5,1361.2,1485,1608.7,1732.5,1856.2,1980,2103.7,2227.4,2351.2,2474.9,2598.7,2722.4,2846.2,2969.9,3093.7,3217.4,3341.2,3464.9,3588.7,3712.4,3836.2,3959.9,4083.7,4207.4,4331.1,4454.9,4578.6,4702.4,4826.1,4949.9,5073.6,5197.4,5321.1,5444.9,5568.6,5692.4,5816.1,5939.9,6063.6,6187.3
      | 0,146.7,293.4,440.1,586.81,733.51,880.21,1026.9,1173.6,1320.3,1467,1613.7,1760.4,1907.1,2053.8,2200.5,2347.2,2493.9,2640.6,2787.3,2934,3080.7,3227.4,3374.1,3520.8,3667.5,3814.2,3960.9,4107.6,4254.3,4401,4547.7,4694.5,4841.2,4987.9,5134.6,5281.3,5428,5574.7,5721.4,5868.1,6014.8,6161.5,6308.2,6454.9,6601.6,6748.3,6895,7041.7,7188.4,7335.1
      | 0,168.44,336.89,505.33,673.78,842.22,1010.7,1179.1,1347.6,1516,1684.4,1852.9,2021.3,2189.8,2358.2,2526.7,2695.1,2863.5,3032,3200.4,3368.9,3537.3,3705.8,3874.2,4042.7,4211.1,4379.5,4548,4716.4,4884.9,5053.3,5221.8,5390.2,5558.6,5727.1,5895.5,6064,6232.4,6400.9,6569.3,6737.8,6906.2,7074.6,7243.1,7411.5,7580,7748.4,7916.9,8085.3,8253.7,8422.2
      | 0,186.02,372.04,558.06,744.08,930.1,1116.1,1302.1,1488.2,1674.2,1860.2,2046.2,2232.2,2418.3,2604.3,2790.3,2976.3,3162.3,3348.4,3534.4,3720.4,3906.4,4092.4,4278.5,4464.5,4650.5,4836.5,5022.5,5208.6,5394.6,5580.6,5766.6,5952.6,6138.7,6324.7,6510.7,6696.7,6882.7,7068.7,7254.8,7440.8,7626.8,7812.8,7998.8,8184.9,8370.9,8556.9,8742.9,8928.9,9115,9301
      | 0,196.87,393.74,590.6,787.47,984.34,1181.2,1378.1,1574.9,1771.8,1968.7,2165.5,2362.4,2559.3,2756.2,2953,3149.9,3346.8,3543.6,3740.5,3937.4,4134.2,4331.1,4528,4724.8,4921.7,5118.6,5315.4,5512.3,5709.2,5906,6102.9,6299.8,6496.6,6693.5,6890.4,7087.2,7284.1,7481,7677.8,7874.7,8071.6,8268.5,8465.3,8662.2,8859.1,9055.9,9252.8,9449.7,9646.5,9843.4
      | 0,199.97,399.95,599.92,799.9,999.87,1199.8,1399.8,1599.8,1799.8,1999.7,2199.7,2399.7,2599.7,2799.6,2999.6,3199.6,3399.6,3599.5,3799.5,3999.5,4199.5,4399.4,4599.4,4799.4,4999.4,5199.3,5399.3,5599.3,5799.2,5999.2,6199.2,6399.2,6599.1,6799.1,6999.1,7199.1,7399,7599,7799,7999,8198.9,8398.9,8598.9,8798.9,8998.8,9198.8,9398.8,9598.8,9798.7,9998.7
      | 0,196.25,392.49,588.74,784.98,981.23,1177.5,1373.7,1570,1766.2,1962.5,2158.7,2354.9,2551.2,2747.4,2943.7,3139.9,3336.2,3532.4,3728.7,3924.9,4121.2,4317.4,4513.6,4709.9,4906.1,5102.4,5298.6,5494.9,5691.1,5887.4,6083.6,6279.9,6476.1,6672.3,6868.6,7064.8,7261.1,7457.3,7653.6,7849.8,8046.1,8242.3,8438.6,8634.8,8831,9027.3,9223.5,9419.8,9616,9812.3
      | 0,187.84,375.67,563.51,751.35,939.18,1127,1314.9,1502.7,1690.5,1878.4,2066.2,2254,2441.9,2629.7,2817.5,3005.4,3193.2,3381.1,3568.9,3756.7,3944.6,4132.4,4320.2,4508.1,4695.9,4883.7,5071.6,5259.4,5447.3,5635.1,5822.9,6010.8,6198.6,6386.4,6574.3,6762.1,6949.9,7137.8,7325.6,7513.5,7701.3,7889.1,8077,8264.8,8452.6,8640.5,8828.3,9016.1,9204,9391.8
      | 0,177.09,354.19,531.28,708.38,885.47,1062.6,1239.7,1416.8,1593.8,1770.9,1948,2125.1,2302.2,2479.3,2656.4,2833.5,3010.6,3187.7,3364.8,3541.9,3719,3896.1,4073.2,4250.3,4427.4,4604.5,4781.5,4958.6,5135.7,5312.8,5489.9,5667,5844.1,6021.2,6198.3,6375.4,6552.5,6729.6,6906.7,7083.8,7260.9,7438,7615.1,7792.1,7969.2,8146.3,8323.4,8500.5,8677.6,8854.7
      | 0,165.86,331.71,497.57,663.43,829.28,995.14,1161,1326.9,1492.7,1658.6,1824.4,1990.3,2156.1,2322,2487.8,2653.7,2819.6,2985.4,3151.3,3317.1,3483,3648.8,3814.7,3980.6,4146.4,4312.3,4478.1,4644,4809.8,4975.7,5141.5,5307.4,5473.3,5639.1,5805,5970.8,6136.7,6302.5,6468.4,6634.3,6800.1,6966,7131.8,7297.7,7463.5,7629.4,7795.2,7961.1,8127,8292.8
      | 0,155.26,310.53,465.79,621.05,776.32,931.58,1086.8,1242.1,1397.4,1552.6,1707.9,1863.2,2018.4,2173.7,2328.9,2484.2,2639.5,2794.7,2950,3105.3,3260.5,3415.8,3571.1,3726.3,3881.6,4036.8,4192.1,4347.4,4502.6,4657.9,4813.2,4968.4,5123.7,5278.9,5434.2,5589.5,5744.7,5900,6055.3,6210.5,6365.8,6521.1,6676.3,6831.6,6986.8,7142.1,7297.4,7452.6,7607.9,7763.2
      | 0,145.88,291.75,437.63,583.5,729.38,875.25,1021.1,1167,1312.9,1458.8,1604.6,1750.5,1896.4,2042.3,2188.1,2334,2479.9,2625.8,2771.6,2917.5,3063.4,3209.3,3355.1,3501,3646.9,3792.8,3938.6,4084.5,4230.4,4376.3,4522.1,4668,4813.9,4959.8,5105.6,5251.5,5397.4,5543.3,5689.1,5835,5980.9,6126.8,6272.6,6418.5,6564.4,6710.3,6856.1,7002,7147.9,7293.8
      | 0,137.87,275.75,413.62,551.49,689.36,827.24,965.11,1103,1240.9,1378.7,1516.6,1654.5,1792.3,1930.2,2068.1,2206,2343.8,2481.7,2619.6,2757.5,2895.3,3033.2,3171.1,3308.9,3446.8,3584.7,3722.6,3860.4,3998.3,4136.2,4274,4411.9,4549.8,4687.7,4825.5,4963.4,5101.3,5239.2,5377,5514.9,5652.8,5790.6,5928.5,6066.4,6204.3,6342.1,6480,6617.9,6755.8,6893.6
      | 0,131.22,262.44,393.66,524.88,656.1,787.32,918.54,1049.8,1181,1312.2,1443.4,1574.6,1705.9,1837.1,1968.3,2099.5,2230.7,2362,2493.2,2624.4,2755.6,2886.8,3018.1,3149.3,3280.5,3411.7,3542.9,3674.2,3805.4,3936.6,4067.8,4199,4330.2,4461.5,4592.7,4723.9,4855.1,4986.3,5117.6,5248.8,5380,5511.2,5642.4,5773.7,5904.9,6036.1,6167.3,6298.5,6429.8,6561]
      MyMap=|
      | [0,1114.7,4367.1,9707.2,17109,26554,38030,51524,67028,84533,1.0403e+05,1.2552e+05,1.4899e+05,1.7444e+05,2.0185e+05,2.3124e+05,2.6259e+05,2.959e+05,3.3117e+05,3.6839e+05,4.0756e+05,4.4868e+05,4.9174e+05,5.3675e+05,5.8369e+05,6.3257e+05,6.8338e+05,7.3613e+05,7.908e+05,8.474e+05,9.0593e+05,9.6638e+05,1.0288e+06,1.093e+06,1.1593e+06,1.2274e+06,1.2974e+06,1.3694e+06,1.4432e+06,1.519e+06,1.5967e+06,1.6763e+06,1.7578e+06,1.8412e+06,1.9265e+06,2.0137e+06,2.1028e+06,2.1938e+06,2.2867e+06,2.3815e+06,2.4782e+06
      | 0,1024.5,4013.8,8921.9,15725,24406,34953,47356,61605,77694,95616,1.1537e+05,1.3694e+05,1.6032e+05,1.8553e+05,2.1254e+05,2.4135e+05,2.7197e+05,3.0438e+05,3.3859e+05,3.7459e+05,4.1238e+05,4.5196e+05,4.9333e+05,5.3647e+05,5.814e+05,6.281e+05,6.7658e+05,7.2683e+05,7.7885e+05,8.3264e+05,8.8821e+05,9.4553e+05,1.0046e+06,1.0655e+06,1.1281e+06,1.1925e+06,1.2586e+06,1.3265e+06,1.3961e+06,1.4675e+06,1.5407e+06,1.6156e+06,1.6922e+06,1.7706e+06,1.8508e+06,1.9327e+06,2.0163e+06,2.1017e+06,2.1889e+06,2.2777e+06
      | 0,938.57,3677,8173.3,14405,22358,32020,43382,56436,71175,87593,1.0568e+05,1.2545e+05,1.4687e+05,1.6996e+05,1.947e+05,2.211e+05,2.4915e+05,2.7884e+05,3.1018e+05,3.4316e+05,3.7778e+05,4.1404e+05,4.5193e+05,4.9146e+05,5.3261e+05,5.754e+05,6.1981e+05,6.6584e+05,7.135e+05,7.6278e+05,8.1368e+05,8.6619e+05,9.2032e+05,9.7607e+05,1.0334e+06,1.0924e+06,1.153e+06,1.2152e+06,1.279e+06,1.3444e+06,1.4114e+06,1.48e+06,1.5502e+06,1.6221e+06,1.6955e+06,1.7705e+06,1.8471e+06,1.9254e+06,2.0052e+06,2.0866e+06
      | 0,856.81,3356.7,7461.3,13151,20411,29231,39603,51520,64974,79962,96478,1.1452e+05,1.3408e+05,1.5515e+05,1.7774e+05,2.0184e+05,2.2744e+05,2.5455e+05,2.8316e+05,3.1327e+05,3.4487e+05,3.7797e+05,4.1256e+05,4.4864e+05,4.8621e+05,5.2527e+05,5.6581e+05,6.0784e+05,6.5134e+05,6.9633e+05,7.4279e+05,7.9073e+05,8.4015e+05,8.9104e+05,9.4341e+05,9.9724e+05,1.0525e+06,1.1093e+06,1.1676e+06,1.2273e+06,1.2885e+06,1.3511e+06,1.4152e+06,1.4808e+06,1.5478e+06,1.6163e+06,1.6862e+06,1.7576e+06,1.8305e+06,1.9048e+06
      | 0,779.25,3052.9,6785.9,11960,18563,26585,36018,46856,59093,72724,87745,1.0415e+05,1.2194e+05,1.4111e+05,1.6165e+05,1.8357e+05,2.0685e+05,2.3151e+05,2.5753e+05,2.8491e+05,3.1365e+05,3.4376e+05,3.7522e+05,4.0803e+05,4.422e+05,4.7772e+05,5.1459e+05,5.5282e+05,5.9238e+05,6.333e+05,6.7556e+05,7.1916e+05,7.641e+05,8.1039e+05,8.5801e+05,9.0697e+05,9.5727e+05,1.0089e+06,1.0619e+06,1.1162e+06,1.1718e+06,1.2288e+06,1.2871e+06,1.3467e+06,1.4077e+06,1.47e+06,1.5336e+06,1.5985e+06,1.6648e+06,1.7324e+06
      | 0,705.9,2765.5,6147.1,10834,16816,24083,32628,42446,53531,65879,79486,94348,1.1046e+05,1.2783e+05,1.4643e+05,1.6629e+05,1.8738e+05,2.0972e+05,2.3329e+05,2.5809e+05,2.8413e+05,3.114e+05,3.399e+05,3.6962e+05,4.0058e+05,4.3276e+05,4.6616e+05,5.0078e+05,5.3662e+05,5.7369e+05,6.1197e+05,6.5146e+05,6.9218e+05,7.3411e+05,7.7725e+05,8.216e+05,8.6717e+05,9.1394e+05,9.6193e+05,1.0111e+06,1.0615e+06,1.1131e+06,1.1659e+06,1.22e+06,1.2752e+06,1.3316e+06,1.3892e+06,1.4481e+06,1.5081e+06,1.5693e+06
      | 0,636.76,2494.6,5545,9773.1,15169,21724,29432,38288,48287,59426,71700,85106,99642,1.153e+05,1.3209e+05,1.5e+05,1.6903e+05,1.8917e+05,2.1044e+05,2.3281e+05,2.563e+05,2.809e+05,3.066e+05,3.3342e+05,3.6134e+05,3.9037e+05,4.205e+05,4.5173e+05,4.8406e+05,5.1749e+05,5.5202e+05,5.8765e+05,6.2438e+05,6.622e+05,7.0111e+05,7.4112e+05,7.8223e+05,8.2442e+05,8.677e+05,9.1208e+05,9.5754e+05,1.0041e+06,1.0517e+06,1.1005e+06,1.1503e+06,1.2012e+06,1.2532e+06,1.3062e+06,1.3604e+06,1.4156e+06
      | 0,571.82,2240.2,4979.5,8776.4,13622,19508,26430,34383,43363,53365,64388,76427,89480,1.0355e+05,1.1862e+05,1.347e+05,1.5179e+05,1.6988e+05,1.8897e+05,2.0907e+05,2.3016e+05,2.5225e+05,2.7534e+05,2.9942e+05,3.2449e+05,3.5056e+05,3.7761e+05,4.0566e+05,4.3469e+05,4.6472e+05,4.9573e+05,5.2772e+05,5.607e+05,5.9467e+05,6.2961e+05,6.6554e+05,7.0245e+05,7.4034e+05,7.7921e+05,8.1906e+05,8.5989e+05,9.017e+05,9.4448e+05,9.8824e+05,1.033e+06,1.0787e+06,1.1254e+06,1.173e+06,1.2216e+06,1.2712e+06
      | 0,511.09,2002.3,4450.7,7844.3,12175,17436,23623,30732,38757,47698,57549,68310,79977,92548,1.0602e+05,1.204e+05,1.3567e+05,1.5184e+05,1.689e+05,1.8686e+05,2.0572e+05,2.2546e+05,2.4609e+05,2.6762e+05,2.9003e+05,3.1332e+05,3.3751e+05,3.6258e+05,3.8853e+05,4.1536e+05,4.4308e+05,4.7167e+05,5.0115e+05,5.3151e+05,5.6274e+05,5.9486e+05,6.2785e+05,6.6171e+05,6.9646e+05,7.3207e+05,7.6857e+05,8.0593e+05,8.4417e+05,8.8328e+05,9.2326e+05,9.6412e+05,1.0058e+06,1.0484e+06,1.0919e+06,1.1362e+06
      | 0,454.56,1780.8,3958.4,6976.8,10828,15508,21011,27333,34471,42422,51185,60755,71132,82313,94296,1.0708e+05,1.2066e+05,1.3505e+05,1.5022e+05,1.662e+05,1.8296e+05,2.0052e+05,2.1888e+05,2.3802e+05,2.5795e+05,2.7867e+05,3.0018e+05,3.2248e+05,3.4556e+05,3.6942e+05,3.9407e+05,4.1951e+05,4.4573e+05,4.7273e+05,5.0051e+05,5.2907e+05,5.5841e+05,5.8853e+05,6.1943e+05,6.5111e+05,6.8356e+05,7.168e+05,7.5081e+05,7.8559e+05,8.2115e+05,8.5749e+05,8.946e+05,9.3248e+05,9.7114e+05,1.0106e+06
      | 0,402.25,1575.9,3502.8,6173.8,9582.1,13723,18592,24187,30503,37540,45293,53762,62945,72839,83443,94756,1.0678e+05,1.195e+05,1.3293e+05,1.4707e+05,1.6191e+05,1.7745e+05,1.9368e+05,2.1062e+05,2.2826e+05,2.466e+05,2.6563e+05,2.8536e+05,3.0578e+05,3.269e+05,3.4872e+05,3.7123e+05,3.9442e+05,4.1832e+05,4.429e+05,4.6817e+05,4.9414e+05,5.2079e+05,5.4814e+05,5.7617e+05,6.0489e+05,6.343e+05,6.6439e+05,6.9517e+05,7.2664e+05,7.588e+05,7.9163e+05,8.2516e+05,8.5937e+05,8.9426e+05
      | 0,354.13,1387.4,3083.9,5435.3,8436,12082,16369,21294,26855,33050,39876,47332,55416,64127,73463,83423,94005,1.0521e+05,1.1703e+05,1.2948e+05,1.4254e+05,1.5622e+05,1.7052e+05,1.8543e+05,2.0096e+05,2.171e+05,2.3386e+05,2.5123e+05,2.6921e+05,2.878e+05,3.0701e+05,3.2682e+05,3.4725e+05,3.6828e+05,3.8993e+05,4.1218e+05,4.3504e+05,4.585e+05,4.8258e+05,5.0725e+05,5.3254e+05,5.5843e+05,5.8493e+05,6.1203e+05,6.3973e+05,6.6804e+05,6.9695e+05,7.2646e+05,7.5658e+05,7.873e+05
      | 0,310.23,1215.4,2701.5,4761.5,7390.2,10584,14339,18654,23526,28952,34932,41464,48546,56176,64355,73080,82351,92166,1.0252e+05,1.1343e+05,1.2487e+05,1.3685e+05,1.4938e+05,1.6244e+05,1.7605e+05,1.9019e+05,2.0487e+05,2.2008e+05,2.3583e+05,2.5212e+05,2.6895e+05,2.863e+05,3.042e+05,3.2262e+05,3.4158e+05,3.6108e+05,3.811e+05,4.0166e+05,4.2275e+05,4.4437e+05,4.6652e+05,4.892e+05,5.1241e+05,5.3615e+05,5.6042e+05,5.8521e+05,6.1054e+05,6.364e+05,6.6278e+05,6.8969e+05
      | 0,270.53,1059.9,2355.8,4152.2,6444.5,9229.4,12504,16267,20515,25247,30462,36158,42334,48988,56120,63728,71813,80372,89405,98911,1.0889e+05,1.1934e+05,1.3026e+05,1.4166e+05,1.5352e+05,1.6585e+05,1.7865e+05,1.9192e+05,2.0566e+05,2.1986e+05,2.3453e+05,2.4967e+05,2.6527e+05,2.8134e+05,2.9787e+05,3.1487e+05,3.3233e+05,3.5026e+05,3.6865e+05,3.875e+05,4.0682e+05,4.266e+05,4.4684e+05,4.6754e+05,4.887e+05,5.1033e+05,5.3241e+05,5.5496e+05,5.7797e+05,6.0143e+05
      | 0,235.04,920.8,2046.8,3607.4,5599,8018.6,10864,14133,17824,21935,26466,31414,36780,42561,48757,55367,62391,69827,77675,85934,94604,1.0368e+05,1.1317e+05,1.2307e+05,1.3338e+05,1.4409e+05,1.5521e+05,1.6674e+05,1.7867e+05,1.9101e+05,2.0376e+05,2.1691e+05,2.3047e+05,2.4443e+05,2.5879e+05,2.7356e+05,2.8873e+05,3.0431e+05,3.2028e+05,3.3666e+05,3.5345e+05,3.7063e+05,3.8821e+05,4.062e+05,4.2459e+05,4.4337e+05,4.6256e+05,4.8215e+05,5.0214e+05,5.2253e+05
      | 0,203.75,798.24,1774.3,3127.2,4853.7,6951.2,9417.7,12252,15451,19015,22943,27233,31884,36896,42267,47997,54086,60533,67336,74496,82011,89882,98108,1.0669e+05,1.1562e+05,1.2491e+05,1.3455e+05,1.4455e+05,1.5489e+05,1.6559e+05,1.7664e+05,1.8804e+05,1.9979e+05,2.1189e+05,2.2434e+05,2.3715e+05,2.503e+05,2.638e+05,2.7765e+05,2.9185e+05,3.064e+05,3.2129e+05,3.3654e+05,3.5213e+05,3.6807e+05,3.8436e+05,4.0099e+05,4.1797e+05,4.353e+05,4.5297e+05
      | 0,176.67,692.15,1538.5,2711.6,4208.6,6027.4,8166.1,10623,13398,16488,19894,23613,27646,31992,36650,41618,46898,52488,58387,64595,71112,77937,85069,92509,1.0026e+05,1.0831e+05,1.1667e+05,1.2533e+05,1.3431e+05,1.4358e+05,1.5316e+05,1.6305e+05,1.7324e+05,1.8373e+05,1.9453e+05,2.0563e+05,2.1703e+05,2.2874e+05,2.4075e+05,2.5306e+05,2.6568e+05,2.7859e+05,2.9181e+05,3.0533e+05,3.1915e+05,3.3327e+05,3.477e+05,3.6242e+05,3.7745e+05,3.9277e+05
      | 0,153.8,602.54,1339.3,2360.6,3663.8,5247,7108.9,9247.9,11663,14353,17318,20556,24067,27850,31905,36230,40826,45692,50828,56232,61905,67847,74056,80533,87277,94287,1.0156e+05,1.0911e+05,1.1692e+05,1.2499e+05,1.3333e+05,1.4194e+05,1.5081e+05,1.5994e+05,1.6934e+05,1.7901e+05,1.8894e+05,1.9913e+05,2.0958e+05,2.203e+05,2.3128e+05,2.4253e+05,2.5403e+05,2.658e+05,2.7783e+05,2.9013e+05,3.0268e+05,3.155e+05,3.2858e+05,3.4192e+05
      | 0,135.13,529.41,1176.8,2074.1,3219.1,4610.2,6246.1,8125.5,10248,12611,15216,18061,21146,24470,28033,31833,35871,40147,44659,49407,54392,59612,65068,70759,76684,82844,89238,95866,1.0273e+05,1.0982e+05,1.1715e+05,1.2471e+05,1.3251e+05,1.4053e+05,1.4879e+05,1.5728e+05,1.66e+05,1.7496e+05,1.8415e+05,1.9356e+05,2.0321e+05,2.1309e+05,2.232e+05,2.3354e+05,2.4411e+05,2.5492e+05,2.6595e+05,2.7721e+05,2.887e+05,3.0042e+05
      | 0,120.67,472.76,1050.9,1852.1,2874.6,4116.9,5577.7,7256.1,9151,11262,13588,16129,18883,21852,25033,28427,32033,35851,39880,44121,48572,53234,58105,63187,68479,73979,79689,85608,91735,98071,1.0462e+05,1.1137e+05,1.1833e+05,1.255e+05,1.3287e+05,1.4045e+05,1.4824e+05,1.5624e+05,1.6444e+05,1.7285e+05,1.8147e+05,1.9029e+05,1.9932e+05,2.0855e+05,2.1799e+05,2.2764e+05,2.3749e+05,2.4755e+05,2.5781e+05,2.6828e+05
      | 0,110.42,432.59,961.56,1694.8,2630.4,3767.1,5103.8,6639.5,8373.5,10305,12433,14758,17279,19995,22906,26012,29311,32805,36492,40372,44445,48710,53168,57818,62660,67694,72918,78334,83941,89738,95727,1.019e+05,1.0827e+05,1.1483e+05,1.2158e+05,1.2852e+05,1.3565e+05,1.4296e+05,1.5047e+05,1.5816e+05,1.6605e+05,1.7412e+05,1.8238e+05,1.9083e+05,1.9947e+05,2.083e+05,2.1731e+05,2.2651e+05,2.359e+05,2.4548e+05
      | 0,120.67,472.76,1050.9,1852.1,2874.6,4116.9,5577.7,7256.1,9151,11262,13588,16129,18883,21852,25033,28427,32033,35851,39880,44121,48572,53234,58105,63187,68479,73979,79689,85608,91735,98071,1.0462e+05,1.1137e+05,1.1833e+05,1.255e+05,1.3287e+05,1.4045e+05,1.4824e+05,1.5624e+05,1.6444e+05,1.7285e+05,1.8147e+05,1.9029e+05,1.9932e+05,2.0855e+05,2.1799e+05,2.2764e+05,2.3749e+05,2.4755e+05,2.5781e+05,2.6828e+05
      | 0,135.13,529.41,1176.8,2074.1,3219.1,4610.2,6246.1,8125.5,10248,12611,15216,18061,21146,24470,28033,31833,35871,40147,44659,49407,54392,59612,65068,70759,76684,82844,89238,95866,1.0273e+05,1.0982e+05,1.1715e+05,1.2471e+05,1.3251e+05,1.4053e+05,1.4879e+05,1.5728e+05,1.66e+05,1.7496e+05,1.8415e+05,1.9356e+05,2.0321e+05,2.1309e+05,2.232e+05,2.3354e+05,2.4411e+05,2.5492e+05,2.6595e+05,2.7721e+05,2.887e+05,3.0042e+05
      | 0,153.8,602.54,1339.3,2360.6,3663.8,5247,7108.9,9247.9,11663,14353,17318,20556,24067,27850,31905,36230,40826,45692,50828,56232,61905,67847,74056,80533,87277,94287,1.0156e+05,1.0911e+05,1.1692e+05,1.2499e+05,1.3333e+05,1.4194e+05,1.5081e+05,1.5994e+05,1.6934e+05,1.7901e+05,1.8894e+05,1.9913e+05,2.0958e+05,2.203e+05,2.3128e+05,2.4253e+05,2.5403e+05,2.658e+05,2.7783e+05,2.9013e+05,3.0268e+05,3.155e+05,3.2858e+05,3.4192e+05
      | 0,176.67,692.15,1538.5,2711.6,4208.6,6027.4,8166.1,10623,13398,16488,19894,23613,27646,31992,36650,41618,46898,52488,58387,64595,71112,77937,85069,92509,1.0026e+05,1.0831e+05,1.1667e+05,1.2533e+05,1.3431e+05,1.4358e+05,1.5316e+05,1.6305e+05,1.7324e+05,1.8373e+05,1.9453e+05,2.0563e+05,2.1703e+05,2.2874e+05,2.4075e+05,2.5306e+05,2.6568e+05,2.7859e+05,2.9181e+05,3.0533e+05,3.1915e+05,3.3327e+05,3.477e+05,3.6242e+05,3.7745e+05,3.9277e+05
      | 0,203.75,798.24,1774.3,3127.2,4853.7,6951.2,9417.7,12252,15451,19015,22943,27233,31884,36896,42267,47997,54086,60533,67336,74496,82011,89882,98108,1.0669e+05,1.1562e+05,1.2491e+05,1.3455e+05,1.4455e+05,1.5489e+05,1.6559e+05,1.7664e+05,1.8804e+05,1.9979e+05,2.1189e+05,2.2434e+05,2.3715e+05,2.503e+05,2.638e+05,2.7765e+05,2.9185e+05,3.064e+05,3.2129e+05,3.3654e+05,3.5213e+05,3.6807e+05,3.8436e+05,4.0099e+05,4.1797e+05,4.353e+05,4.5297e+05
      | 0,235.04,920.8,2046.8,3607.4,5599,8018.6,10864,14133,17824,21935,26466,31414,36780,42561,48757,55367,62391,69827,77675,85934,94604,1.0368e+05,1.1317e+05,1.2307e+05,1.3338e+05,1.4409e+05,1.5521e+05,1.6674e+05,1.7867e+05,1.9101e+05,2.0376e+05,2.1691e+05,2.3047e+05,2.4443e+05,2.5879e+05,2.7356e+05,2.8873e+05,3.0431e+05,3.2028e+05,3.3666e+05,3.5345e+05,3.7063e+05,3.8821e+05,4.062e+05,4.2459e+05,4.4337e+05,4.6256e+05,4.8215e+05,5.0214e+05,5.2253e+05
      | 0,270.53,1059.9,2355.8,4152.2,6444.5,9229.4,12504,16267,20515,25247,30462,36158,42334,48988,56120,63728,71813,80372,89405,98911,1.0889e+05,1.1934e+05,1.3026e+05,1.4166e+05,1.5352e+05,1.6585e+05,1.7865e+05,1.9192e+05,2.0566e+05,2.1986e+05,2.3453e+05,2.4967e+05,2.6527e+05,2.8134e+05,2.9787e+05,3.1487e+05,3.3233e+05,3.5026e+05,3.6865e+05,3.875e+05,4.0682e+05,4.266e+05,4.4684e+05,4.6754e+05,4.887e+05,5.1033e+05,5.3241e+05,5.5496e+05,5.7797e+05,6.0143e+05
      | 0,310.23,1215.4,2701.5,4761.5,7390.2,10584,14339,18654,23526,28952,34932,41464,48546,56176,64355,73080,82351,92166,1.0252e+05,1.1343e+05,1.2487e+05,1.3685e+05,1.4938e+05,1.6244e+05,1.7605e+05,1.9019e+05,2.0487e+05,2.2008e+05,2.3583e+05,2.5212e+05,2.6895e+05,2.863e+05,3.042e+05,3.2262e+05,3.4158e+05,3.6108e+05,3.811e+05,4.0166e+05,4.2275e+05,4.4437e+05,4.6652e+05,4.892e+05,5.1241e+05,5.3615e+05,5.6042e+05,5.8521e+05,6.1054e+05,6.364e+05,6.6278e+05,6.8969e+05
      | 0,354.13,1387.4,3083.9,5435.3,8436,12082,16369,21294,26855,33050,39876,47332,55416,64127,73463,83423,94005,1.0521e+05,1.1703e+05,1.2948e+05,1.4254e+05,1.5622e+05,1.7052e+05,1.8543e+05,2.0096e+05,2.171e+05,2.3386e+05,2.5123e+05,2.6921e+05,2.878e+05,3.0701e+05,3.2682e+05,3.4725e+05,3.6828e+05,3.8993e+05,4.1218e+05,4.3504e+05,4.585e+05,4.8258e+05,5.0725e+05,5.3254e+05,5.5843e+05,5.8493e+05,6.1203e+05,6.3973e+05,6.6804e+05,6.9695e+05,7.2646e+05,7.5658e+05,7.873e+05
      | 0,402.25,1575.9,3502.8,6173.8,9582.1,13723,18592,24187,30503,37540,45293,53762,62945,72839,83443,94756,1.0678e+05,1.195e+05,1.3293e+05,1.4707e+05,1.6191e+05,1.7745e+05,1.9368e+05,2.1062e+05,2.2826e+05,2.466e+05,2.6563e+05,2.8536e+05,3.0578e+05,3.269e+05,3.4872e+05,3.7123e+05,3.9442e+05,4.1832e+05,4.429e+05,4.6817e+05,4.9414e+05,5.2079e+05,5.4814e+05,5.7617e+05,6.0489e+05,6.343e+05,6.6439e+05,6.9517e+05,7.2664e+05,7.588e+05,7.9163e+05,8.2516e+05,8.5937e+05,8.9426e+05
      | 0,454.56,1780.8,3958.4,6976.8,10828,15508,21011,27333,34471,42422,51185,60755,71132,82313,94296,1.0708e+05,1.2066e+05,1.3505e+05,1.5022e+05,1.662e+05,1.8296e+05,2.0052e+05,2.1888e+05,2.3802e+05,2.5795e+05,2.7867e+05,3.0018e+05,3.2248e+05,3.4556e+05,3.6942e+05,3.9407e+05,4.1951e+05,4.4573e+05,4.7273e+05,5.0051e+05,5.2907e+05,5.5841e+05,5.8853e+05,6.1943e+05,6.5111e+05,6.8356e+05,7.168e+05,7.5081e+05,7.8559e+05,8.2115e+05,8.5749e+05,8.946e+05,9.3248e+05,9.7114e+05,1.0106e+06
      | 0,511.09,2002.3,4450.7,7844.3,12175,17436,23623,30732,38757,47698,57549,68310,79977,92548,1.0602e+05,1.204e+05,1.3567e+05,1.5184e+05,1.689e+05,1.8686e+05,2.0572e+05,2.2546e+05,2.4609e+05,2.6762e+05,2.9003e+05,3.1332e+05,3.3751e+05,3.6258e+05,3.8853e+05,4.1536e+05,4.4308e+05,4.7167e+05,5.0115e+05,5.3151e+05,5.6274e+05,5.9486e+05,6.2785e+05,6.6171e+05,6.9646e+05,7.3207e+05,7.6857e+05,8.0593e+05,8.4417e+05,8.8328e+05,9.2326e+05,9.6412e+05,1.0058e+06,1.0484e+06,1.0919e+06,1.1362e+06
      | 0,571.82,2240.2,4979.5,8776.4,13622,19508,26430,34383,43363,53365,64388,76427,89480,1.0355e+05,1.1862e+05,1.347e+05,1.5179e+05,1.6988e+05,1.8897e+05,2.0907e+05,2.3016e+05,2.5225e+05,2.7534e+05,2.9942e+05,3.2449e+05,3.5056e+05,3.7761e+05,4.0566e+05,4.3469e+05,4.6472e+05,4.9573e+05,5.2772e+05,5.607e+05,5.9467e+05,6.2961e+05,6.6554e+05,7.0245e+05,7.4034e+05,7.7921e+05,8.1906e+05,8.5989e+05,9.017e+05,9.4448e+05,9.8824e+05,1.033e+06,1.0787e+06,1.1254e+06,1.173e+06,1.2216e+06,1.2712e+06
      | 0,636.76,2494.6,5545,9773.1,15169,21724,29432,38288,48287,59426,71700,85106,99642,1.153e+05,1.3209e+05,1.5e+05,1.6903e+05,1.8917e+05,2.1044e+05,2.3281e+05,2.563e+05,2.809e+05,3.066e+05,3.3342e+05,3.6134e+05,3.9037e+05,4.205e+05,4.5173e+05,4.8406e+05,5.1749e+05,5.5202e+05,5.8765e+05,6.2438e+05,6.622e+05,7.0111e+05,7.4112e+05,7.8223e+05,8.2442e+05,8.677e+05,9.1208e+05,9.5754e+05,1.0041e+06,1.0517e+06,1.1005e+06,1.1503e+06,1.2012e+06,1.2532e+06,1.3062e+06,1.3604e+06,1.4156e+06
      | 0,705.9,2765.5,6147.1,10834,16816,24083,32628,42446,53531,65879,79486,94348,1.1046e+05,1.2783e+05,1.4643e+05,1.6629e+05,1.8738e+05,2.0972e+05,2.3329e+05,2.5809e+05,2.8413e+05,3.114e+05,3.399e+05,3.6962e+05,4.0058e+05,4.3276e+05,4.6616e+05,5.0078e+05,5.3662e+05,5.7369e+05,6.1197e+05,6.5146e+05,6.9218e+05,7.3411e+05,7.7725e+05,8.216e+05,8.6717e+05,9.1394e+05,9.6193e+05,1.0111e+06,1.0615e+06,1.1131e+06,1.1659e+06,1.22e+06,1.2752e+06,1.3316e+06,1.3892e+06,1.4481e+06,1.5081e+06,1.5693e+06
      | 0,779.25,3052.9,6785.9,11960,18563,26585,36018,46856,59093,72724,87745,1.0415e+05,1.2194e+05,1.4111e+05,1.6165e+05,1.8357e+05,2.0685e+05,2.3151e+05,2.5753e+05,2.8491e+05,3.1365e+05,3.4376e+05,3.7522e+05,4.0803e+05,4.422e+05,4.7772e+05,5.1459e+05,5.5282e+05,5.9238e+05,6.333e+05,6.7556e+05,7.1916e+05,7.641e+05,8.1039e+05,8.5801e+05,9.0697e+05,9.5727e+05,1.0089e+06,1.0619e+06,1.1162e+06,1.1718e+06,1.2288e+06,1.2871e+06,1.3467e+06,1.4077e+06,1.47e+06,1.5336e+06,1.5985e+06,1.6648e+06,1.7324e+06
      | 0,856.81,3356.7,7461.3,13151,20411,29231,39603,51520,64974,79962,96478,1.1452e+05,1.3408e+05,1.5515e+05,1.7774e+05,2.0184e+05,2.2744e+05,2.5455e+05,2.8316e+05,3.1327e+05,3.4487e+05,3.7797e+05,4.1256e+05,4.4864e+05,4.8621e+05,5.2527e+05,5.6581e+05,6.0784e+05,6.5134e+05,6.9633e+05,7.4279e+05,7.9073e+05,8.4015e+05,8.9104e+05,9.4341e+05,9.9724e+05,1.0525e+06,1.1093e+06,1.1676e+06,1.2273e+06,1.2885e+06,1.3511e+06,1.4152e+06,1.4808e+06,1.5478e+06,1.6163e+06,1.6862e+06,1.7576e+06,1.8305e+06,1.9048e+06
      | 0,938.57,3677,8173.3,14405,22358,32020,43382,56436,71175,87593,1.0568e+05,1.2545e+05,1.4687e+05,1.6996e+05,1.947e+05,2.211e+05,2.4915e+05,2.7884e+05,3.1018e+05,3.4316e+05,3.7778e+05,4.1404e+05,4.5193e+05,4.9146e+05,5.3261e+05,5.754e+05,6.1981e+05,6.6584e+05,7.135e+05,7.6278e+05,8.1368e+05,8.6619e+05,9.2032e+05,9.7607e+05,1.0334e+06,1.0924e+06,1.153e+06,1.2152e+06,1.279e+06,1.3444e+06,1.4114e+06,1.48e+06,1.5502e+06,1.6221e+06,1.6955e+06,1.7705e+06,1.8471e+06,1.9254e+06,2.0052e+06,2.0866e+06
      | 0,1024.5,4013.8,8921.9,15725,24406,34953,47356,61605,77694,95616,1.1537e+05,1.3694e+05,1.6032e+05,1.8553e+05,2.1254e+05,2.4135e+05,2.7197e+05,3.0438e+05,3.3859e+05,3.7459e+05,4.1238e+05,4.5196e+05,4.9333e+05,5.3647e+05,5.814e+05,6.281e+05,6.7658e+05,7.2683e+05,7.7885e+05,8.3264e+05,8.8821e+05,9.4553e+05,1.0046e+06,1.0655e+06,1.1281e+06,1.1925e+06,1.2586e+06,1.3265e+06,1.3961e+06,1.4675e+06,1.5407e+06,1.6156e+06,1.6922e+06,1.7706e+06,1.8508e+06,1.9327e+06,2.0163e+06,2.1017e+06,2.1889e+06,2.2777e+06
      | 0,1114.7,4367.1,9707.2,17109,26554,38030,51524,67028,84533,1.0403e+05,1.2552e+05,1.4899e+05,1.7444e+05,2.0185e+05,2.3124e+05,2.6259e+05,2.959e+05,3.3117e+05,3.6839e+05,4.0756e+05,4.4868e+05,4.9174e+05,5.3675e+05,5.8369e+05,6.3257e+05,6.8338e+05,7.3613e+05,7.908e+05,8.474e+05,9.0593e+05,9.6638e+05,1.0288e+06,1.093e+06,1.1593e+06,1.2274e+06,1.2974e+06,1.3694e+06,1.4432e+06,1.519e+06,1.5967e+06,1.6763e+06,1.7578e+06,1.8412e+06,1.9265e+06,2.0137e+06,2.1028e+06,2.1938e+06,2.2867e+06,2.3815e+06,2.4782e+06]
      settings: LibrarySourceBlock=vehdynlibtire/Longitudinal Wheel - No Brake
  Wheelbase : Constant  Value=2.5
  XPosIntegrator : Integrator  InitialCondition=18
  XPosScope : Scope
  YPosInteg : Integrator
  YPosScope : Scope
  ZeroPhi : Constant  Value=0
  powergui : spspowerguiLib/powergui  Priority=1  SimulationMode=Discrete  SampleTime=1e-6  frequency=60  Iterations=50  frequencyindice=0  Pbase=100e6  ErrMax=1e-4  UnitsV=kV  UnitsW=MW  buscounter=0  FunctionMessages=off  echomessages=off  EnableUseOfTLC=off  CurrentSourceSwitches=off  DisableSnubberDevices=off  DisableRonSwitches=off  DisableVfSwitches=off  DisplayEquations=off  AutomaticDiscreteSolvers=off  SolverType=Tustin/Backward Euler (TBE)  Interpol=off  ExternalGateDelay=off  methode=off  Ts=100  x0status=blocks  SPID=on  SwTol=0  HookPort=off  NonlinearTolerance=1e-4  nMaxIteration=100  ContinueOnMaxIteration=off  RestoreLinks=warning  ResistiveCurrentMeasurement=off  Frange=[0:2:500]  Ylog=off  Xlog=on  ShowGrid=off  save=off  variable=ZData  structure=0  ZoomFFT=off  StartTime=0.0  cycles=1  DisplayStyle=1  fundamental=60  FreqAxis=off  MaxFrequency=1000  frequencyindicesteady=1  RmsSteady=1  display=off
  wires:
  PWM1/1 -> Inv1/1
  BL1/1 -> Inv1/2
  Wh1/3 -> Sat2/1
  MATLAB Function2/1(XVelocity) -> XPosIntegrator/1
  MATLAB Function2/4(TrailerOrientationChange) -> TlrOrientInteg/1
  Wh1/2 -> FrontForceSum/1
  FrontForceSum/1 -> CarBody/2
  VelGain1/1 -> Sat4/1
  VelSum/1 -> VelDelay/1
  XPosIntegrator/1 -> XPosScope/1, MATLAB Function/1(x_c)
  Wheelbase/1 -> MATLAB Function/6(L_c)
  LookaheadDist/1 -> MATLAB Function/5(L_d)
  VelDelay/1 -> VelError/2, CarBody/5, VelOffset/2, TrailerBody/1, Wh1/2
  PhiCalc/1 -> RelativeAngleScope/1, PhiError/2
  StrngSum/1 -> StrngLimiter/1
  VRefSwitch/1 -> VelError/1
  PhiSwitch/1 -> PhiError/1
  PhiError/1 -> HitchPID/1
  HitchPID/1 -> HitchSwitch/1
  ZeroPhi/1 -> HitchSwitch/2
  HitchSwitch/1 -> StrngSum/2
  VelError/1 -> VelPID/1
  FwR/1 -> CarBody/3
  Constant1/1 -> VarRes1/1
  DCMot1/1 -> BusSelector1/1
  BusSelector1/1 -> Wh1/1  "<Electrical torque Te (n m)>"
  Constant3/1 -> VarCap1/1
  VelPID/1 -> VelPIDSat/1
  ModGain/1 -> Sat1/1
  Sat1/1 -> PWM1/1
  TL1/1 -> DCMot1/1
  MATLAB Function3/1(Fz) -> Wh1/3
  VelOffset/1 -> MATLAB Function2/1(CarVelocity)
  VellOffsetConst/1 -> VelOffset/1
  MATLAB Function3/2(Fh) -> CarBody/4
  Sat2/1 -> VelGain1/1
  VelPIDSat/1 -> ModGain/1
  TlrOrientInteg/1 -> TrlDelay/1
  Sat4/1 -> VelSum/1
  TrlDelay/1 -> TrailerOrientationScope/1, PhiCalc/2, MATLAB Function2/4(TrailerOrientation)
  YPosInteg/1 -> MATLAB Function/2(y_c), YPosScope/1
  VRefParking/1 -> VRefSwitch/2
  VRefStraight/1 -> VRefSwitch/3
  VRefReverse/1 -> VRefSwitch/4
  TrajReverse/1 -> TrajRefSwitch/4
  TrajStraight/1 -> TrajRefSwitch/3
  TrajRefSwitch/1 -> MATLAB Function/4(ref_traj)
  TrajParking/1 -> TrajRefSwitch/2
  PhiRefParking/1 -> PhiSwitch/2
  PhiRefReverse/1 -> PhiSwitch/4
  PhiRefStraight/1 -> PhiSwitch/3
  TrailerEnable/1 -> MATLAB Function2/5(TrailerEnable), MATLAB Function3/1(TrailerEnable)
  ManSelect/1 -> MATLAB Function/7(manselect), MATLAB Function2/6(manselect), MATLAB Function1/1(manselect)
  MATLAB Function1/1(port_index) -> TrajRefSwitch/1, PhiSwitch/1, VRefSwitch/1
  MATLAB Function/1(delta) -> Abs/1
  StrngLimiter/1 -> Gain2/1, CarBody/1
  CarOrientInteg/1 -> CarOrientationScope/1, MATLAB Function2/3(CarOrientation), MATLAB Function/3(theta_c), PhiCalc/1
  MATLAB Function2/2(YVelocity) -> Gain1/1
  MATLAB Function2/3(CarOrientationChange) -> Gain/1
  Gain/1 -> CarOrientInteg/1
  Gain1/1 -> YPosInteg/1
  Gain2/1 -> MATLAB Function2/2(SteeringAngle)
  Abs/1 -> StrngSum/1
  connections:
  Inv1/LConn2 -- DCMot1/RConn1
  Batt/LConn2 -- Ground1/LConn1 -- DCMot1/RConn2
  Batt/LConn1 -- VarCap1/LConn1 -- DCMot1/LConn2 -- VarRes1/LConn1
  VarRes1/RConn1 -- VarCap1/RConn1 -- Inv1/LConn1 -- DCMot1/LConn1
